simulink model "punto5_daAaB"  (R2023a)
settings: Solver=VariableStepAuto  StartTime=0.0  StopTime=2000  RelTol=1e-3
values from neighbouring files (symbols this model uses):
  Pn1 = 100e6    (= 100000000)    [punto5_codice.m]
  Pn2 = 50e6    (= 50000000)    [punto5_codice.m]
  tau1 = 10    [punto5_codice.m]
  tau2 = 5    [punto5_codice.m]
libraries: simulink x2
settings Model: Creator=marco  LastModifiedBy=Samsung
settings OptimizationCC: ReuseModelBlockBuffer=off

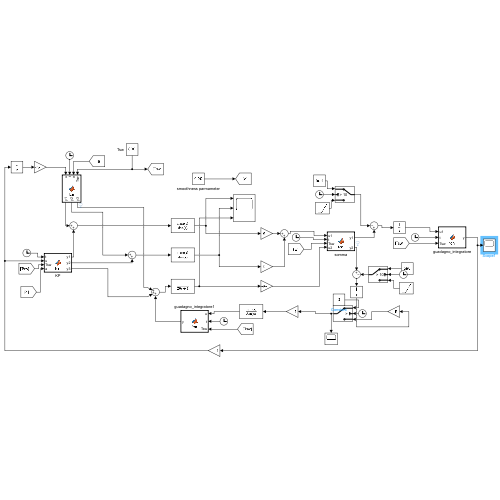
[thumbnail: Simulink's stored preview of the top-level diagram]
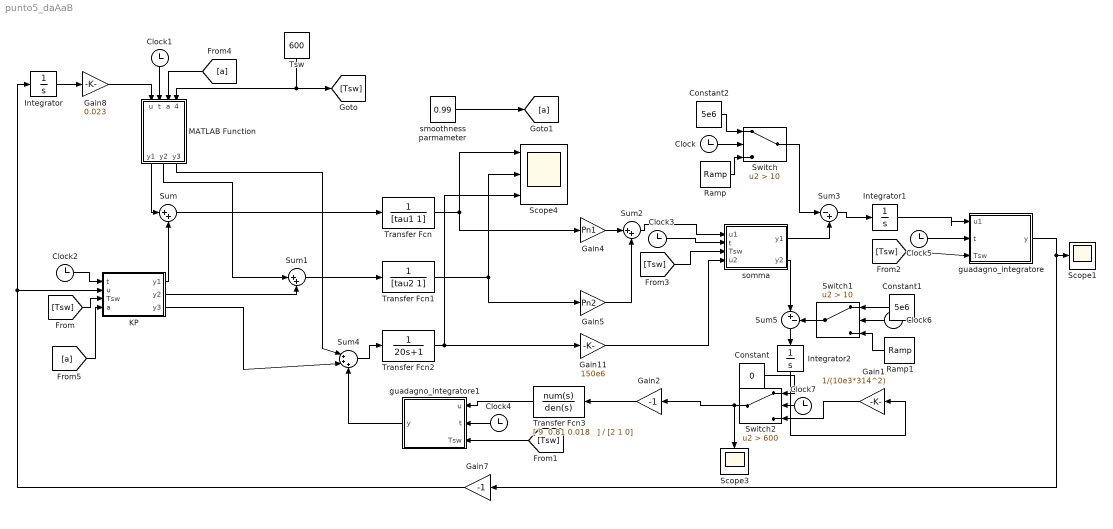
== system punto5_daAaB ==
  Clock{,1..7} (8 alike) : Clock
  Constant : Constant  Value=0
  Constant1 : Constant  Value=5e6
  Constant2 : Constant  Value=5e6
  Gain1 : Gain  Gain=1/(10e3*314^2)
  Gain11 : Gain  Gain=150e6
  Gain2 : Gain  Gain=-1
  Gain4 : Gain  Gain=Pn1
  Gain5 : Gain  Gain=Pn2
  Gain7 : Gain  Gain=-1
  Gain8 : Gain  Gain=0.023
  Integrator : Integrator
  Integrator1 : Integrator
  Integrator2 : Integrator
  KP : MATLAB Function  TreatAsAtomicUnit=on
  MATLAB Function : MATLAB Function  TreatAsAtomicUnit=on
  Ramp : simulink/Sources/Ramp  slope=500000  start=0  InitialOutput=0
  Ramp1 : simulink/Sources/Ramp  slope=500000  start=0  InitialOutput=0
  Scope1 : Scope
  Scope3 : Scope
  Scope4 : Scope  NumInputPorts=3
  Sum : Sum  Inputs=|++
  Sum1 : Sum  Inputs=|++
  Sum2 : Sum  Inputs=|++
  Sum3 : Sum  Inputs=|-+
  Sum4 : Sum  Inputs=|+++
  Sum5 : Sum  Inputs=|+-
  Switch : Switch  Criteria=u2 > Threshold  Threshold=10  SaturateOnIntegerOverflow=off  InputSameDT=off
  Switch1 : Switch  Criteria=u2 > Threshold  Threshold=10  SaturateOnIntegerOverflow=off  InputSameDT=off
  Switch2 : Switch  Criteria=u2 > Threshold  Threshold=600  SaturateOnIntegerOverflow=off  InputSameDT=off
  Transfer Fcn : TransferFcn  Denominator=[tau1 1]
  Transfer Fcn1 : TransferFcn  Denominator=[tau2 1]
  Transfer Fcn2 : TransferFcn  Denominator=[20 1]
  Transfer Fcn3 : TransferFcn  Numerator="[ 9  0.81 0.018   ]"  Denominator=[2 1 0]
  Tsw : Constant  Value=600
  guadagno_integratore : MATLAB Function  TreatAsAtomicUnit=on
  guadagno_integratore1 : MATLAB Function  TreatAsAtomicUnit=on
  smoothness parmameter : Constant  Value=0.99
  somma : MATLAB Function  TreatAsAtomicUnit=on
  wires:
  Sum2/1 -> somma/1(u1)
  Integrator1/1 -> guadagno_integratore/1(u1)
  Ramp/1 -> Switch/3
  Gain4/1 -> Sum2/1
  Switch/1 -> Sum3/1
  KP/2(y2) -> Sum1/2
  Transfer Fcn/1 -> Gain4/1, Scope4/1
  Transfer Fcn1/1 -> Gain5/1, Scope4/2
  Gain7/1 -> Integrator/1, KP/2(u)
  Integrator/1 -> Gain8/1
  Clock/1 -> Switch/2
  guadagno_integratore/1(y) -> Scope1/1, Gain7/1
  Gain8/1 -> MATLAB Function/1(u)
  Constant2/1 -> Switch/1
  Transfer Fcn2/1 -> Gain11/1, Scope4/3
  Sum3/1 -> Integrator1/1
  Sum1/1 -> Transfer Fcn1/1
  Sum/1 -> Transfer Fcn/1
  Gain5/1 -> Sum2/2
  Gain11/1 -> somma/4(u2)
  KP/1(y1) -> Sum/2
  Clock1/1 -> MATLAB Function/2(t)
  Clock2/1 -> KP/1(t)
  Clock3/1 -> somma/2(t)
  Integrator2/1 -> Gain1/1
  Gain2/1 -> Transfer Fcn3/1
  Clock4/1 -> guadagno_integratore1/2(t)
  Transfer Fcn3/1 -> guadagno_integratore1/1(u)
  guadagno_integratore1/1(y) -> Sum4/3
  MATLAB Function/3(y3) -> Sum4/1
  Sum4/1 -> Transfer Fcn2/1
  Clock5/1 -> guadagno_integratore/2(t)
  Switch1/1 -> Sum5/2
  Ramp1/1 -> Switch1/3
  Clock6/1 -> Switch1/2
  somma/2(y2) -> Sum5/1
  Sum5/1 -> Integrator2/1
  MATLAB Function/1(y1) -> Sum/1
  KP/3(y3) -> Sum4/2
  MATLAB Function/2(y2) -> Sum1/1
  Tsw/1 -> MATLAB Function/4(Tsw), [Tsw]
  [Tsw] -> KP/3(Tsw)
  [Tsw] -> guadagno_integratore1/3(Tsw)
  [Tsw] -> guadagno_integratore/3(Tsw)
  [Tsw] -> somma/3(Tsw)
  smoothness parmameter/1 -> [a]
  [a] -> MATLAB Function/3(a)
  [a] -> KP/4(a)
  somma/1(y1) -> Sum3/2
  Constant1/1 -> Switch1/1
  Switch2/1 -> Gain2/1, Scope3/1
  Gain1/1 -> Switch2/3
  Constant/1 -> Switch2/1
  Clock7/1 -> Switch2/2

== matlab function punto5_daAaB/KP ==
  data: t input; u input; y1 output; y2 output; y3 output; Tsw input; a input
function [y1, y2,y3] = fcn( t, u, Tsw, a)
if t>Tsw
    y1=(0.91*(1-a^(t-Tsw))+0.014*a^(t-Tsw))*u;   
    y2=(4.773*(1-a^(t-Tsw))+3.686*a^(t-Tsw))*u;
    y3=(0.182*(1-a^(t-Tsw)))*u;
else 
    y1=0.014*u;
    y2=3.686*u;
    y3=0;
end

== matlab function punto5_daAaB/MATLAB Function ==
  data: u input; y1 output; t input; a input; y2 output; y3 output; Tsw input
function [y1, y2,y3] = fcn(u, t, a, Tsw)
 if t>Tsw
    y1=(0.4*(1-a^(t-Tsw))+1/3*a^(t-Tsw))*u;
    y2=(0.2*(1-a^(t-Tsw))+2/3*a^(t-Tsw))*u;
    y3=(0.4*(1-a^(t-Tsw)))*u;
  else 
    y1=1/3*u;
    y2=2/3*u;
    y3=0;
 
end

== matlab function punto5_daAaB/somma ==
  data: u1 input; t input; Tsw input; u2 input; y1 output; y2 output
function [y1, y2] = fcn(u1, t, Tsw, u2)
if t>Tsw
    y1=(u1+u2); 
    y2=0;
else 
    y1=u1; 
    y2=u2;
end

== matlab function punto5_daAaB/guadagno_integratore ==
  data: u1 input; y output; t input; Tsw input
function y = fcn(u1, t, Tsw)
if t>Tsw
    y=1/(40e3*314^2)*u1;
else 
    y=1/(30e3*314^2)*u1; 
end

== matlab function punto5_daAaB/guadagno_integratore1 ==
  data: u input; y output; t input; Tsw input
function y = fcn(u,t,Tsw)
if t>Tsw
    y=0;
else 
    y=u; 
end
